simulink library "DriftControllerLibrary"  (R2014a)
settings: Solver=ode45  StartTime=0.0  StopTime=10.0  RelTol=1e-3
values from neighbouring files (symbols this model uses):
  alpha_lookup = alpha_sl:-0.001:-1*alpha_sl    [Fyf_lookup_table.m]
  alpha_prm = 0.9    [InitMap.m]
  beta_prm = 1    [InitMap.m]
  curve_prm = curve_prm.data    [InitMap.m]
  discrete_prm = discrete_prm.data    [InitMap.m]
  errLim_prm = 0.005    [InitMap.m]
  Fyf_lookup_2W = -Cf*tan(alpha_lookup) + Cf^2*(2 - mu_s_assumed_f/mu_p_assumed_f)*abs(tan(alpha_lookup)).*tan(alpha_lookup)/(3*mu_p_assumed_f*Fzf) -      Cf^3*tan(alpha_lookup).^3*(1-2*mu_s_assumed_f/(3*mu_p_assumed_f))/(9*mu_p_assumed_f^2*Fzf^2)    [Fyf_lookup_table.m]
  Fyf_lookup_4W = -(Cf/2)*tan(alpha_lookup) + (Cf/2)^2*(2 - mu_s_assumed_f/mu_p_assumed_f)*abs(tan(alpha_lookup)).*tan(alpha_lookup)/(3*mu_p_assumed_f*(Fzf/2)) -      (Cf/2)^3*tan(alpha_lookup).^3*(1-2*mu_s_assumed_f/(3*mu_p_assumed_f))/(9*mu_p_assumed_f^2*(Fzf/2)^2)    [Fyf_lookup_table.m]
  iterLim_prm = 30    [InitMap.m]
  map_prm = map_prm.data    [InitMap.m]
  numTerms_prm = 10    [InitMap.m]
  seg_prm = seg_prm.data    [InitMap.m]
  Ts = 0.002    [DSC_Control_Analysis.m]    (also in DSC_Control_Analysis_Exp.m; DSC_Speed_Control_Analysis.m; EC_params_nissan.m; Ext_MPCPara.m = SSD.Ts)
  useZ_prm = 0    [InitMap.m]
undefined symbols (not defined in the file or in its folder): ack, axInit, beta_vec, betaDes, betaThreshold, delta_sol, deltaLimits, Feasible, Fxr_sol, FxrEq, Fyf_sat, Fyf_sol, Kbeta, Kr, KUx, KUx_Drift, mu_p_assumed, mu_s_assumed, param, r_vec, rThreshold, sr, steering_limit, tau_DK, tau_DSC, tHold, tLimits, Ux_vec, UxEq, UxLimits, VoltsToTorque, VoltsToTorqueRegen, wc
libraries: DriftControllerLibrary x2, simulink x1
(part 1 of 2)
settings Model: Creator=Administrator  LastModifiedBy=cbeal

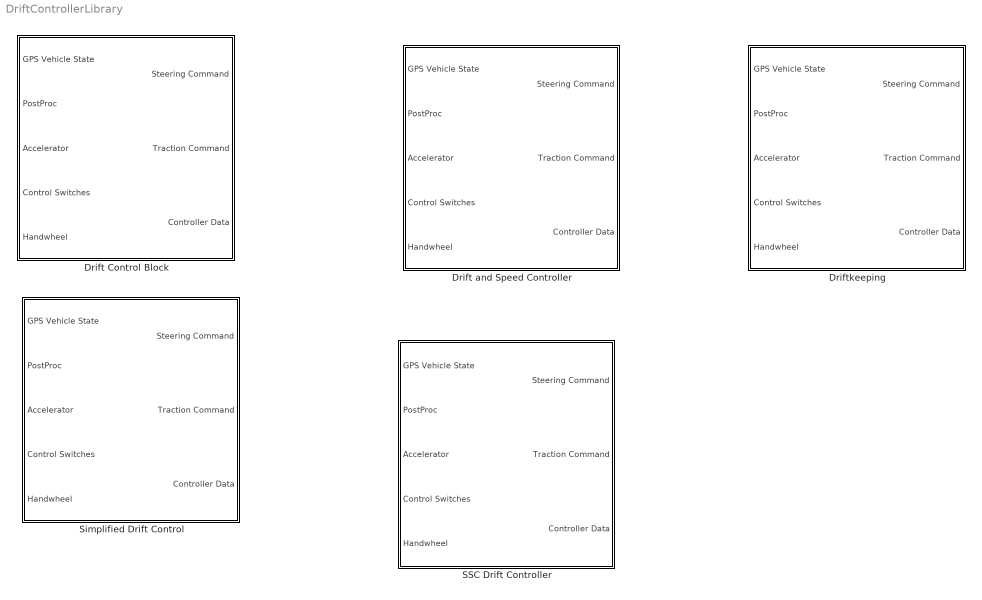
== system DriftControllerLibrary ==
  Drift Control Block : Subsystem  mask(Drift Controller Options){CoordinationEnable=on, UseGalvez=off, CoordType=Exact}
      mask prompts: CoordinationEnable "Use Longitudinal Coordination"; UseGalvez "Use Galvez Test Sequence"; CoordType "Coordination Method"
      mask init:
      | p1_params;
      | drift_params_DSC;
      | Fyf_lookup_table;
      | SteeringController;
      | 
      | coordinationswitch = [gcs '/Drift Control Block' '/Drift Controller Subsystem' '/Use Longitudinal Coordination'];
      | galvezswitch = [gcs '/Drift Control Block' '/Drift Controller Subsystem' '/Use Galvez Test Sequence'];
      | coordtypeswitch = [gcs '/Drift Control Block' '/Drift Controller Subsystem' '/Coordination Method'];
      | % NLObserverswitch = [gcs '/Nonlinear Observer' '/Enable Observer'];
      | % NLObserverStorageswitch = [gcs '/Nonlinear Observer' '/Enable Observer Estimate Storage'];
      | 
      | % default settings
      | set_param(coordinationswitch, 'value', '0');
      | set_param(galvezswitch, 'value', '0');
      | % set_param(NLObserverswitch, 'value', '1');
      | % set_param(NLObserverStorageswitch, 'value', '1'); 
      | 
      | %Look at checkbox to see if longitudinal coordination is desired
      | if (CoordinationEnable == 1)
      |     set_param(coordinationswitch, 'value', '1');
      | end
      | 
      | %Look at checkbox to see if Galvez test sequence is set
      | if (UseGalvez == 1)
      |     set_param(galvezswitch, 'value', '1');
      | end
      | 
      | %Look at popup menu to determine what coordination method to use
      | if (CoordType == 1)
      |     set_param(coordtypeswitch, 'value', '1');
      | elseif (CoordType == 2)
      |     set_param(coordtypeswitch, 'value', '2');
      | end
      mask TypeOptions CoordType: Linearization | Exact
  Drift and Speed Controller : Subsystem  mask(Drift Controller Options){UseGalvez=off}
      mask prompts: UseGalvez "Use Galvez Test Sequence"
      mask init:
      | p1_params;
      | drift_params_DSC_Speed;
      | SteeringController;
      | Fyf_lookup_table;
      | LoadDSCControlMap;
      | 
      | galvezswitch = [gcs '/Drift and Speed Controller' '/Drift Controller Subsystem' ...
      |     '/Use Galvez Test Sequence'];
      | 
      | % default settings
      | set_param(galvezswitch, 'value', '0');
      | 
      | %Look at checkbox to see if Galvez test sequence is set
      | if (UseGalvez == 1)
      |     set_param(galvezswitch, 'value', '1');
      | end
  Driftkeeping : Subsystem  mask(Drift Controller Options){}
      mask init:
      | p1_params;
      | driftkeeping_params;
      | Fyf_lookup_table;
      | SteeringController;
      | InitMap;
  SSC Drift Controller : Subsystem  mask(Drift Controller Options){UseGalvez=off}
      mask prompts: UseGalvez "Use Galvez Test Sequence"
      mask init:
      | p1_params;
      | drift_params_SSC;
      | SteeringController;
      | 
      | galvezswitch = [gcs '/SSC Drift Controller' '/SSC Drift Controller Subsystem' '/Use Galvez Test Sequence'];
      | % NLObserverswitch = [gcs '/Nonlinear Observer' '/Enable Observer'];
      | % NLObserverStorageswitch = [gcs '/Nonlinear Observer' '/Enable Observer Estimate Storage'];
      | 
      | % default settings
      | set_param(galvezswitch, 'value', '0');
      | % set_param(NLObserverswitch, 'value', '1');
      | % set_param(NLObserverStorageswitch, 'value', '1'); 
      | 
      | %Look at checkbox to see if Galvez test sequence is set
      | if (UseGalvez == 1)
      |     set_param(galvezswitch, 'value', '1');
      | end
  Simplified Drift Control : Subsystem  mask(Drift Controller Options){CoordinationEnable=Fxr, UseGalvez=off}
      mask prompts: CoordinationEnable "Use Longitudinal Coordination"; UseGalvez "Use Galvez Test Sequence"
      mask init:
      | p1_params;
      | drift_params_SDSC;
      | Fyf_lookup_table;
      | SteeringController;
      | 
      | coordinationswitch = [gcs '/Simplified Drift Control' '/Drift Controller Subsystem' '/Use Longitudinal Coordination'];
      | galvezswitch = [gcs '/Simplified Drift Control' '/Drift Controller Subsystem' '/Use Galvez Test Sequence'];
      | differentialswitch = [gcs '/Simplified Drift Control' '/Drift Controller Subsystem' '/Use Differential Drive'];
      | % NLObserverswitch = [gcs '/Nonlinear Observer' '/Enable Observer'];
      | % NLObserverStorageswitch = [gcs '/Nonlinear Observer' '/Enable Observer Estimate Storage'];
      | 
      | % default settings
      | set_param(coordinationswitch, 'value', '0');
      | set_param(galvezswitch, 'value', '0');
      | set_param(differentialswitch, 'value', '0');
      | % set_param(NLObserverswitch, 'value', '1');
      | % set_param(NLObserverStorageswitch, 'value', '1'); 
      | 
      | %Look at checkbox to see if longitudinal coordination is desired
      | if (CoordinationEnable == 2)
      |     set_param(coordinationswitch, 'value', '1');
      | end
      | 
      | if (CoordinationEnable == 3)
      |     set_param(differentialswitch, 'value', '1');
      | end
      | 
      | 
      | %Look at checkbox to see if Galvez test sequence is set
      | if (UseGalvez == 1)
      |     set_param(galvezswitch, 'value', '1');
      | end
      mask TypeOptions CoordinationEnable: None | Fxr | M_diff

== system DriftControllerLibrary/Drift Control Block ==
  GPS Vehicle State : Inport
  PostProc : Inport  Port=2
  Accelerator : Inport  Port=3
  Control Switches : Inport  Port=4
  Handwheel : Inport  Port=5
  Bus Selector1 : BusSelector  OutputSignals=Cruise Control Switch,Auto-Steer Switch,Brake Pedal Signal
  Drift Controller Subsystem : Subsystem
  Enable Logic : Subsystem
  Logical Operator : Logic  AllPortsSameDT=off  OutDataTypeStr=boolean
  Steering Command : Outport
  Traction Command : Outport  Port=2
  Controller Data : Outport  Port=3
  wires:
  Drift Controller Subsystem/3(Traction Command (A)) -> Traction Command/1
  Drift Controller Subsystem/2("Steering Command (rad, roadwheels)") -> Steering Command/1
  Drift Controller Subsystem/1(Controller Data) -> Controller Data/1
  Handwheel/1 -> Drift Controller Subsystem/3(Handwheel Angle)
  Accelerator/1 -> Drift Controller Subsystem/4(Go Pedal)
  GPS Vehicle State/1 -> Drift Controller Subsystem/2(GPS Vehicle State)
  PostProc/1 -> Drift Controller Subsystem/5(PostProc)
  Control Switches/1 -> Bus Selector1/1
  Enable Logic/1(Enable) -> Drift Controller Subsystem/1(Enable)
  Bus Selector1/1 -> Logical Operator/1  "<Cruise Control Switch>"
  Bus Selector1/2 -> Logical Operator/2  "<Auto-Steer Switch>"
  Bus Selector1/3 -> Enable Logic/2(Brake Pedal)  "<Brake Pedal Signal>"
  Logical Operator/1 -> Enable Logic/1(Enable Command)

== system DriftControllerLibrary/Drift and Speed Controller ==
  GPS Vehicle State : Inport
  PostProc : Inport  Port=2
  Accelerator : Inport  Port=3
  Control Switches : Inport  Port=4
  Handwheel : Inport  Port=5
  Bus Selector1 : BusSelector  OutputSignals=Cruise Control Switch,Auto-Steer Switch,Brake Pedal Signal
  Drift Controller Subsystem : Subsystem
  Enable Logic : Subsystem
  Logical Operator : Logic  AllPortsSameDT=off  OutDataTypeStr=boolean
  Steering Command : Outport
  Traction Command : Outport  Port=2
  Controller Data : Outport  Port=3
  wires:
  Logical Operator/1 -> Enable Logic/1(Enable Command)
  Bus Selector1/3 -> Enable Logic/2(Brake Pedal)  "<Brake Pedal Signal>"
  Bus Selector1/2 -> Logical Operator/2  "<Auto-Steer Switch>"
  Bus Selector1/1 -> Logical Operator/1  "<Cruise Control Switch>"
  Enable Logic/1(Enable) -> Drift Controller Subsystem/1(Enable)
  Control Switches/1 -> Bus Selector1/1
  PostProc/1 -> Drift Controller Subsystem/5(PostProc)
  GPS Vehicle State/1 -> Drift Controller Subsystem/2(GPS Vehicle State)
  Accelerator/1 -> Drift Controller Subsystem/4(Go Pedal)
  Handwheel/1 -> Drift Controller Subsystem/3(Handwheel Angle)
  Drift Controller Subsystem/1(Controller Data) -> Controller Data/1
  Drift Controller Subsystem/2("Steering Command (rad, roadwheels)") -> Steering Command/1
  Drift Controller Subsystem/3(Traction Command (A)) -> Traction Command/1

== system DriftControllerLibrary/Driftkeeping ==
  GPS Vehicle State : Inport
  PostProc : Inport  Port=2
  Accelerator : Inport  Port=3
  Control Switches : Inport  Port=4
  Handwheel : Inport  Port=5
  Bus Selector1 : BusSelector  OutputSignals=Cruise Control Switch,Auto-Steer Switch,Brake Pedal Signal
  Driftkeeping Subsystem : Subsystem
  Enable Logic : Subsystem
  Logical Operator : Logic  AllPortsSameDT=off  OutDataTypeStr=boolean
  Steering Command : Outport
  Traction Command : Outport  Port=2
  Controller Data : Outport  Port=3
  wires:
  Logical Operator/1 -> Enable Logic/1(Enable Command)
  Bus Selector1/3 -> Enable Logic/2(Brake Pedal)  "<Brake Pedal Signal>"
  Bus Selector1/2 -> Logical Operator/2  "<Auto-Steer Switch>"
  Bus Selector1/1 -> Logical Operator/1  "<Cruise Control Switch>"
  Enable Logic/1(Enable) -> Driftkeeping Subsystem/1(Enable)
  Control Switches/1 -> Bus Selector1/1
  PostProc/1 -> Driftkeeping Subsystem/5(PostProc)
  GPS Vehicle State/1 -> Driftkeeping Subsystem/2(GPS Vehicle State)
  Accelerator/1 -> Driftkeeping Subsystem/4(Go Pedal)
  Handwheel/1 -> Driftkeeping Subsystem/3(Handwheel Angle)
  Driftkeeping Subsystem/1(Controller Data) -> Controller Data/1
  Driftkeeping Subsystem/2("Steering Command (rad, roadwheels)") -> Steering Command/1
  Driftkeeping Subsystem/3(Traction Command (A)) -> Traction Command/1

== system DriftControllerLibrary/SSC Drift Controller ==
  GPS Vehicle State : Inport
  PostProc : Inport  Port=2
  Accelerator : Inport  Port=3
  Control Switches : Inport  Port=4
  Handwheel : Inport  Port=5
  Bus Selector1 : BusSelector  OutputSignals=Cruise Control Switch,Auto-Steer Switch,Brake Pedal Signal
  Enable Logic : Subsystem
  Logical Operator : Logic  AllPortsSameDT=off  OutDataTypeStr=boolean
  SSC Drift Controller Subsystem : Subsystem
  Terminator : Terminator
  Steering Command : Outport
  Traction Command : Outport  Port=2
  Controller Data : Outport  Port=3
  wires:
  Logical Operator/1 -> Enable Logic/1(Enable Command)
  Bus Selector1/3 -> Enable Logic/2(Brake Pedal)  "<Brake Pedal Signal>"
  Bus Selector1/2 -> Logical Operator/2  "<Auto-Steer Switch>"
  Bus Selector1/1 -> Logical Operator/1  "<Cruise Control Switch>"
  Enable Logic/1(Enable) -> SSC Drift Controller Subsystem/1(Enable)
  Control Switches/1 -> Bus Selector1/1
  GPS Vehicle State/1 -> SSC Drift Controller Subsystem/2(GPS Vehicle State)
  Accelerator/1 -> SSC Drift Controller Subsystem/4(Go Pedal)
  Handwheel/1 -> SSC Drift Controller Subsystem/3(Handwheel Angle)
  SSC Drift Controller Subsystem/1(Controller Data) -> Controller Data/1
  SSC Drift Controller Subsystem/2("Steering Command (rad, roadwheels)") -> Steering Command/1
  SSC Drift Controller Subsystem/3(Traction Command (A)) -> Traction Command/1
  PostProc/1 -> Terminator/1

== system DriftControllerLibrary/Simplified Drift Control ==
  GPS Vehicle State : Inport
  PostProc : Inport  Port=2
  Accelerator : Inport  Port=3
  Control Switches : Inport  Port=4
  Handwheel : Inport  Port=5
  Bus Selector1 : BusSelector  OutputSignals=Cruise Control Switch,Auto-Steer Switch,Brake Pedal Signal
  Drift Controller Subsystem : Subsystem
  Enable Logic : Subsystem
  Logical Operator : Logic  AllPortsSameDT=off  OutDataTypeStr=boolean
  Steering Command : Outport
  Traction Command : Outport  Port=2
  Controller Data : Outport  Port=3
  wires:
  Drift Controller Subsystem/3(Traction Command (A)) -> Traction Command/1
  Drift Controller Subsystem/2("Steering Command (rad, roadwheels)") -> Steering Command/1
  Drift Controller Subsystem/1(Controller Data) -> Controller Data/1
  Handwheel/1 -> Drift Controller Subsystem/3(Handwheel Angle)
  Accelerator/1 -> Drift Controller Subsystem/4(Go Pedal)
  GPS Vehicle State/1 -> Drift Controller Subsystem/2(GPS Vehicle State)
  PostProc/1 -> Drift Controller Subsystem/5(PostProc)
  Control Switches/1 -> Bus Selector1/1
  Enable Logic/1(Enable) -> Drift Controller Subsystem/1(Enable)
  Bus Selector1/1 -> Logical Operator/1  "<Cruise Control Switch>"
  Bus Selector1/2 -> Logical Operator/2  "<Auto-Steer Switch>"
  Bus Selector1/3 -> Enable Logic/2(Brake Pedal)  "<Brake Pedal Signal>"
  Logical Operator/1 -> Enable Logic/1(Enable Command)

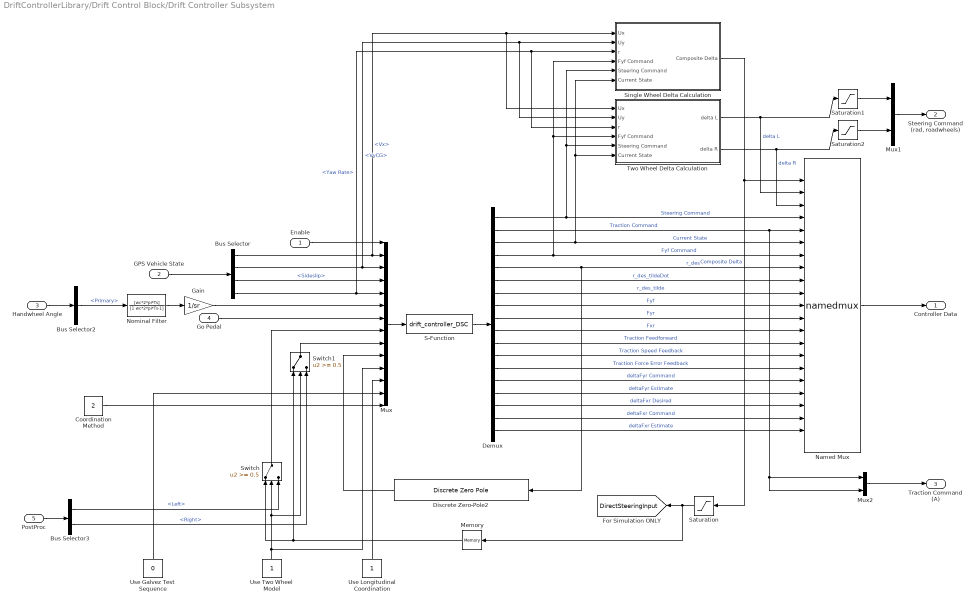
== system DriftControllerLibrary/Drift Control Block/Drift Controller Subsystem ==
  Enable : Inport
  GPS Vehicle State : Inport  Port=2
  Handwheel Angle : Inport  Port=3
  Go Pedal : Inport  Port=4
  PostProc : Inport  Port=5
  Bus Selector : BusSelector  OutputSignals=Vx,VyCG,Sideslip,Yaw Rate
  Bus Selector2 : BusSelector  OutputSignals=Primary
  Bus Selector3 : BusSelector  OutputSignals=Steer Angles.Left,Steer Angles.Right
  Coordination Method : Constant  Value=2
  Demux : Demux  Outputs=18
  Discrete Zero-Pole2 : DiscreteZeroPole  Zeros=[]  Poles=[exp(-Ts/tau_DSC)]  Gain=1-exp(-Ts/tau_DSC)  SampleTime=Ts
  Gain : Gain  Gain=1/sr
  Memory : Memory
  Mux : Mux  Inputs=14
  Mux1 : Mux  Inputs=2
  Mux2 : Mux  Inputs=2
  Named Mux : S-Function  FunctionName=namedmux  Parameters=inputcount,inputsizes  EnableBusSupport=off  mask{fname=datadescDriftController}
      mask prompts: fname "Data description function name"
      mask help:
      | Combines input signals into a single output vector, according to a structure that provides the names and sizes of each signal.
      |
      | The parameter below should be set to the name of a function which returns a 1xN structure array, where N is the number of input signals.  The structure should contain fields "size" which specifies the width of the input signal, and "name" which specifies its name.
      mask init:
      | desc=eval(fname);
      | %if(class(desc)~='cell')
      | %	error('Incorrect description');
      | %end
      | inputcount=length(desc);
      | if((inputcount<1)|(inputcount>50))
      | 	error('Inappropriate number of inputs.');
      | end
      | 
      | inputsizes=[desc.size];
      | 
      | x=min(inputcount*ones(1,50),1:50);
      mask Display:
      | port_label('input',x(1),desc(x(1)).name);
      | port_label('input',x(2),desc(x(2)).name);
      | port_label('input',x(3),desc(x(3)).name);
      | port_label('input',x(4),desc(x(4)).name);
      | port_label('input',x(5),desc(x(5)).name);
      | port_label('input',x(6),desc(x(6)).name);
      | port_label('input',x(7),desc(x(7)).name);
      | port_label('input',x(8),desc(x(8)).name);
      | port_label('input',x(9),desc(x(9)).name);
      | port_label('input',x(10),desc(x(10)).name);
      | port_label('input',x(11),desc(x(11)).name);
      | port_label('input',x(12),desc(x(12)).name);
      | port_label('input',x(13),desc(x(13)).name);
      | port_label('input',x(14),desc(x(14)).name);
      | port_label('input',x(15),desc(x(15)).name);
      | port_label('input',x(16),desc(x(16)).name);
      | port_label('input',x(17),desc(x(17)).name);
      | port_label('input',x(18),desc(x(18)).name);
      | port_label('input',x(19),desc(x(19)).name);
      | port_label('input',x(20),desc(x(20)).name);
      | port_label('input',x(21),desc(x(21)).name);
      | port_label('input',x(22),desc(x(22)).name);
      | port_label('input',x(23),desc(x(23)).name);
      | port_label('input',x(24),desc(x(24)).name);
      | port_label('input',x(25),desc(x(25)).name);
      | port_label('input',x(26),desc(x(26)).name);
      | port_label('input',x(27),desc(x(27)).name);
      | port_label('input',x(28),desc(x(28)).name);
      | port_label('input',x(29),desc(x(29)).name);
      | port_label('input',x(30),desc(x(30)).name);
  Nominal Filter : DiscreteFilter  Numerator=[wc*2*pi*Ts]  Denominator=[1 wc*2*pi*Ts-1]  SampleTime=Ts
  S-Function : S-Function  FunctionName=drift_controller_DSC  Parameters=axInit,tHold,UxLimits,deltaLimits,tLimits,betaThreshold,rThreshold,betaDes,UxEq,FxrEq,Kbeta,Kr,KUx,KUx_Drift,tau_DSC,VoltsToTorque,VoltsToTorqueRegen,param.drive_ratio,param.rl.r,param.m,param.Iz,param.a,param.b,param.c,param.fl.C,param.fr.C,param.rl.C,param.rr.C,mu_p_assumed,mu_s_assumed,Fyf_sat,Ts  EnableBusSupport=off
  Saturation : Saturate  UpperLimit=steering_limit*pi/180  LowerLimit=-steering_limit*pi/180
  Saturation1 : Saturate  UpperLimit=steering_limit*pi/180  LowerLimit=-steering_limit*pi/180
  Saturation2 : Saturate  UpperLimit=steering_limit*pi/180  LowerLimit=-steering_limit*pi/180
  Single Wheel Delta Calculation : Subsystem
  Switch : Switch  Threshold=0.5
  Switch1 : Switch  Threshold=0.5
  Two Wheel Delta Calculation : Subsystem
  Use Galvez Test Sequence : Constant  Value=0
  Use Longitudinal Coordination : Constant
  Use Two Wheel Model : Constant
  Controller Data : Outport
  "Steering Command (rad, roadwheels)" : Outport  Port=2
  Traction Command (A) : Outport  Port=3
  tag scope: DirectSteeringInput=global
  wires:
  Coordination Method/1 -> Mux/14
  Mux2/1 -> Traction Command (A)/1
  Nominal Filter/1 -> Gain/1
  Bus Selector2/1 -> Nominal Filter/1  "<Primary>"
  Demux/14 -> Named Mux/17  "deltaFyr Command"
  Single Wheel Delta Calculation/1(Composite Delta) -> Saturation/1, Named Mux/1  "Composite Delta"
  Demux/1 -> Single Wheel Delta Calculation/5(Steering Command), Two Wheel Delta Calculation/5(Steering Command), Named Mux/4  "Steering Command"
  Demux/2 -> Mux2/2, Mux2/1, Named Mux/5  "Traction Command"
  Demux/3 -> Single Wheel Delta Calculation/6(Current State), Two Wheel Delta Calculation/6(Current State), Named Mux/6  "Current State"
  Demux/5 -> Discrete Zero-Pole2/1, Named Mux/8  "r_des"
  Demux/4 -> Single Wheel Delta Calculation/4(Fyf Command), Two Wheel Delta Calculation/4(Fyf Command), Named Mux/7  "Fyf Command"
  Named Mux/1 -> Controller Data/1
  Demux/18 -> Named Mux/21  "deltaFxr Estimate"
  Demux/17 -> Named Mux/20  "deltaFxr Command"
  Demux/16 -> Named Mux/19  "deltaFxr Desired"
  Demux/15 -> Named Mux/18  "deltaFyr Estimate"
  Demux/13 -> Named Mux/16  "Traction Force Error Feedback"
  Demux/12 -> Named Mux/15  "Traction Speed Feedback"
  Demux/11 -> Named Mux/14  "Traction Feedforward"
  Demux/10 -> Named Mux/13  "Fxr"
  Demux/9 -> Named Mux/12  "Fyr"
  Demux/8 -> Named Mux/11  "Fyf"
  Demux/7 -> Named Mux/10  "r_des_tilde"
  Demux/6 -> Named Mux/9  "r_des_tildeDot"
  Two Wheel Delta Calculation/2(delta R) -> Named Mux/3, Saturation2/1  "delta R"
  Saturation2/1 -> Mux1/2
  Saturation1/1 -> Mux1/1
  Mux1/1 -> "Steering Command (rad, roadwheels)"/1
  Enable/1 -> Mux/1
  Use Galvez Test Sequence/1 -> Mux/13
  Use Longitudinal Coordination/1 -> Mux/12
  Discrete Zero-Pole2/1 -> Mux/10
  Switch1/1 -> Mux/9
  Switch/1 -> Mux/8
  Use Two Wheel Model/1 -> Mux/11, Switch/2, Switch1/2
  Bus Selector3/2 -> Switch1/3  "<Right>"
  Bus Selector3/1 -> Switch/3  "<Left>"
  Memory/1 -> Switch1/1, Switch/1
  Two Wheel Delta Calculation/1(delta L) -> Named Mux/2, Saturation1/1  "delta L"
  Saturation/1 -> Memory/1, [DirectSteeringInput]
  PostProc/1 -> Bus Selector3/1
  Bus Selector/4 -> Two Wheel Delta Calculation/3(r), Single Wheel Delta Calculation/3(r), Mux/5  "<Yaw Rate>"
  Bus Selector/3 -> Mux/4  "<Sideslip>"
  Bus Selector/2 -> Two Wheel Delta Calculation/2(Uy), Single Wheel Delta Calculation/2(Uy), Mux/3  "<VyCG>"
  Gain/1 -> Mux/6
  Go Pedal/1 -> Mux/7
  Mux/1 -> S-Function/1
  Bus Selector/1 -> Two Wheel Delta Calculation/1(Ux), Single Wheel Delta Calculation/1(Ux), Mux/2  "<Vx>"
  S-Function/1 -> Demux/1
  Handwheel Angle/1 -> Bus Selector2/1
  GPS Vehicle State/1 -> Bus Selector/1

== system DriftControllerLibrary/Drift Control Block/Enable Logic ==
  Enable Command : Inport
  Brake Pedal : Inport  Port=2
  Delay : Subsystem
  Latch1 : Subsystem  TreatAsAtomicUnit=on
  Logical Operator : Logic  Operator=OR  AllPortsSameDT=off  OutDataTypeStr=float('double')
  Logical Operator1 : Logic  AllPortsSameDT=off  OutDataTypeStr=float('double')
  Logical Operator2 : Logic  Operator=NOT  AllPortsSameDT=off  OutDataTypeStr=float('double')
  Enable : Outport
  wires:
  Logical Operator2/1 -> Logical Operator1/2
  Logical Operator1/1 -> Latch1/1(In1)
  Logical Operator/1 -> Latch1/Trigger
  Brake Pedal/1 -> Logical Operator/2, Logical Operator2/1
  Delay/1(Out) -> Logical Operator/1
  Enable Command/1 -> Logical Operator1/1, Delay/1(In)
  Latch1/1(Out1) -> Enable/1

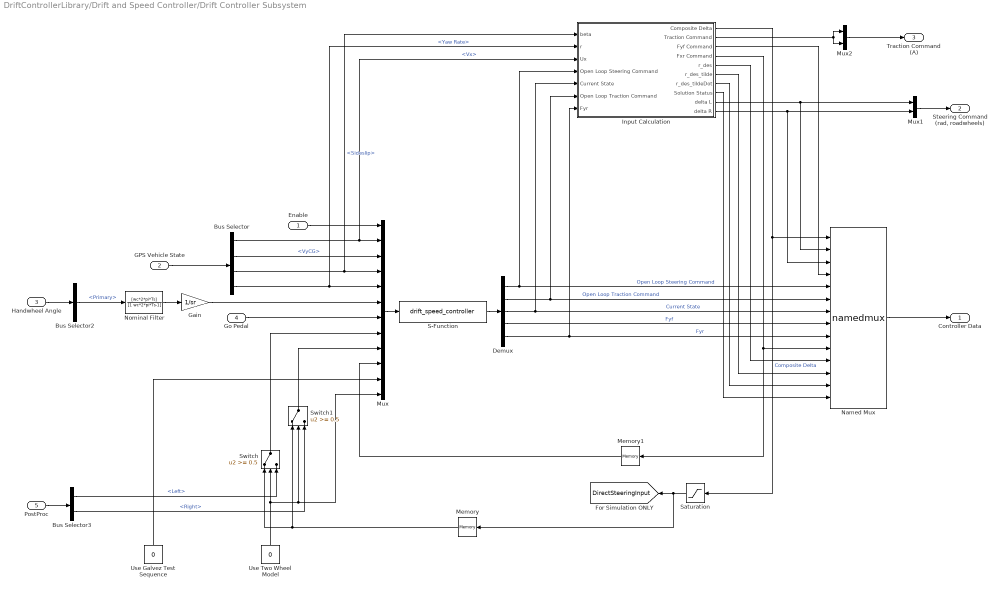
== system DriftControllerLibrary/Drift and Speed Controller/Drift Controller Subsystem ==
  Enable : Inport
  GPS Vehicle State : Inport  Port=2
  Handwheel Angle : Inport  Port=3
  Go Pedal : Inport  Port=4
  PostProc : Inport  Port=5
  Bus Selector : BusSelector  OutputSignals=Vx,VyCG,Sideslip,Yaw Rate
  Bus Selector2 : BusSelector  OutputSignals=Primary
  Bus Selector3 : BusSelector  OutputSignals=Steer Angles.Left,Steer Angles.Right
  Demux : Demux  Outputs=5
  Gain : Gain  Gain=1/sr
  Input Calculation : Subsystem
  Memory : Memory
  Memory1 : Memory
  Mux : Mux  Inputs=12
  Mux1 : Mux  Inputs=2
  Mux2 : Mux  Inputs=2
  Named Mux : S-Function  FunctionName=namedmux  Parameters=inputcount,inputsizes  EnableBusSupport=off  mask{fname=datadescDriftSpeedController}
      mask prompts: fname "Data description function name"
      mask help:
      | Combines input signals into a single output vector, according to a structure that provides the names and sizes of each signal.
      |
      | The parameter below should be set to the name of a function which returns a 1xN structure array, where N is the number of input signals.  The structure should contain fields "size" which specifies the width of the input signal, and "name" which specifies its name.
      mask init: same as DriftControllerLibrary/Drift Control Block/Drift Controller Subsystem/Named Mux
      mask Display:
      | port_label('input',x(1),desc(x(1)).name);
      | port_label('input',x(2),desc(x(2)).name);
      | port_label('input',x(3),desc(x(3)).name);
      | port_label('input',x(4),desc(x(4)).name);
      | port_label('input',x(5),desc(x(5)).name);
      | port_label('input',x(6),desc(x(6)).name);
      | port_label('input',x(7),desc(x(7)).name);
      | port_label('input',x(8),desc(x(8)).name);
      | port_label('input',x(9),desc(x(9)).name);
      | port_label('input',x(10),desc(x(10)).name);
      | port_label('input',x(11),desc(x(11)).name);
      | port_label('input',x(12),desc(x(12)).name);
      | port_label('input',x(13),desc(x(13)).name);
      | port_label('input',x(14),desc(x(14)).name);
      | port_label('input',x(15),desc(x(15)).name);
      | port_label('input',x(16),desc(x(16)).name);
      | port_label('input',x(17),desc(x(17)).name);
      | port_label('input',x(18),desc(x(18)).name);
      | port_label('input',x(19),desc(x(19)).name);
      | port_label('input',x(20),desc(x(20)).name);
      | port_label('input',x(21),desc(x(21)).name);
      | port_label('input',x(22),desc(x(22)).name);
      | port_label('input',x(23),desc(x(23)).name);
      | port_label('input',x(24),desc(x(24)).name);
      | port_label('input',x(25),desc(x(25)).name);
      | port_label('input',x(26),desc(x(26)).name);
      | port_label('input',x(27),desc(x(27)).name);
      | port_label('input',x(28),desc(x(28)).name);
      | port_label('input',x(29),desc(x(29)).name);
      | port_label('input',x(30),desc(x(30)).name);
  Nominal Filter : DiscreteFilter  Numerator=[wc*2*pi*Ts]  Denominator=[1 wc*2*pi*Ts-1]  SampleTime=Ts
  S-Function : S-Function  FunctionName=drift_speed_controller  Parameters=axInit,tHold,UxLimits,deltaLimits,tLimits, KUx, betaThreshold,rThreshold,VoltsToTorque,VoltsToTorqueRegen,param.drive_ratio,param.rl.r,param.m,param.Iz,param.a,param.b,param.c,param.fl.C,param.fr.C,param.rl.C,param.rr.C,mu_p_assumed,mu_s_assumed,Ts  EnableBusSupport=off
  Saturation : Saturate  UpperLimit=steering_limit*pi/180  LowerLimit=-steering_limit*pi/180
  Switch : Switch  Threshold=0.5
  Switch1 : Switch  Threshold=0.5
  Use Galvez Test Sequence : Constant  Value=0
  Use Two Wheel Model : Constant  Value=0
  Controller Data : Outport
  "Steering Command (rad, roadwheels)" : Outport  Port=2
  Traction Command (A) : Outport  Port=3
  tag scope: DirectSteeringInput=global
  wires:
  GPS Vehicle State/1 -> Bus Selector/1
  Handwheel Angle/1 -> Bus Selector2/1
  Bus Selector/1 -> Mux/2, Input Calculation/3(Ux)  "<Vx>"
  Mux/1 -> S-Function/1
  Go Pedal/1 -> Mux/7
  Gain/1 -> Mux/6
  Bus Selector/2 -> Mux/3  "<VyCG>"
  Bus Selector/3 -> Mux/4, Input Calculation/1(beta)  "<Sideslip>"
  Bus Selector/4 -> Mux/5, Input Calculation/2(r)  "<Yaw Rate>"
  PostProc/1 -> Bus Selector3/1
  Saturation/1 -> [DirectSteeringInput], Memory/1
  Memory/1 -> Switch/1, Switch1/1
  Bus Selector3/1 -> Switch/3  "<Left>"
  Bus Selector3/2 -> Switch1/3  "<Right>"
  Use Two Wheel Model/1 -> Switch/2, Switch1/2, Mux/12
  Switch/1 -> Mux/8
  Switch1/1 -> Mux/9
  Enable/1 -> Mux/1
  Mux1/1 -> "Steering Command (rad, roadwheels)"/1
  Named Mux/1 -> Controller Data/1
  Demux/3 -> Input Calculation/5(Current State), Named Mux/7  "Current State"
  Input Calculation/1(Composite Delta) -> Saturation/1, Named Mux/1  "Composite Delta"
  Bus Selector2/1 -> Nominal Filter/1  "<Primary>"
  Nominal Filter/1 -> Gain/1
  Demux/2 -> Input Calculation/6(Open Loop Traction Command), Named Mux/6  "Open Loop Traction Command"
  Mux2/1 -> Traction Command (A)/1
  Input Calculation/2(Traction Command) -> Mux2/1, Mux2/2
  S-Function/1 -> Demux/1
  Demux/1 -> Named Mux/5, Input Calculation/4(Open Loop Steering Command)  "Open Loop Steering Command"
  Input Calculation/3(Fyf Command) -> Named Mux/4
  Demux/4 -> Named Mux/8  "Fyf"
  Demux/5 -> Named Mux/9, Input Calculation/7(Fyr)  "Fyr"
  Input Calculation/5(r_des) -> Named Mux/11
  Input Calculation/6(r_des_tilde) -> Named Mux/12
  Input Calculation/7(r_des_tildeDot) -> Named Mux/13
  Input Calculation/4(Fxr Command) -> Named Mux/10, Memory1/1
  Input Calculation/8(Solution Status) -> Named Mux/14
  Use Galvez Test Sequence/1 -> Mux/11
  Memory1/1 -> Mux/10
  Input Calculation/9(delta L) -> Named Mux/2, Mux1/1
  Input Calculation/10(delta R) -> Named Mux/3, Mux1/2

== system DriftControllerLibrary/Drift and Speed Controller/Enable Logic ==
  Enable Command : Inport
  Brake Pedal : Inport  Port=2
  Delay : Subsystem
  Latch1 : Subsystem  TreatAsAtomicUnit=on
  Logical Operator : Logic  Operator=OR  AllPortsSameDT=off  OutDataTypeStr=float('double')
  Logical Operator1 : Logic  AllPortsSameDT=off  OutDataTypeStr=float('double')
  Logical Operator2 : Logic  Operator=NOT  AllPortsSameDT=off  OutDataTypeStr=float('double')
  Enable : Outport
  wires:
  Latch1/1(Out1) -> Enable/1
  Enable Command/1 -> Delay/1(In), Logical Operator1/1
  Delay/1(Out) -> Logical Operator/1
  Brake Pedal/1 -> Logical Operator2/1, Logical Operator/2
  Logical Operator/1 -> Latch1/Trigger
  Logical Operator1/1 -> Latch1/1(In1)
  Logical Operator2/1 -> Logical Operator1/2

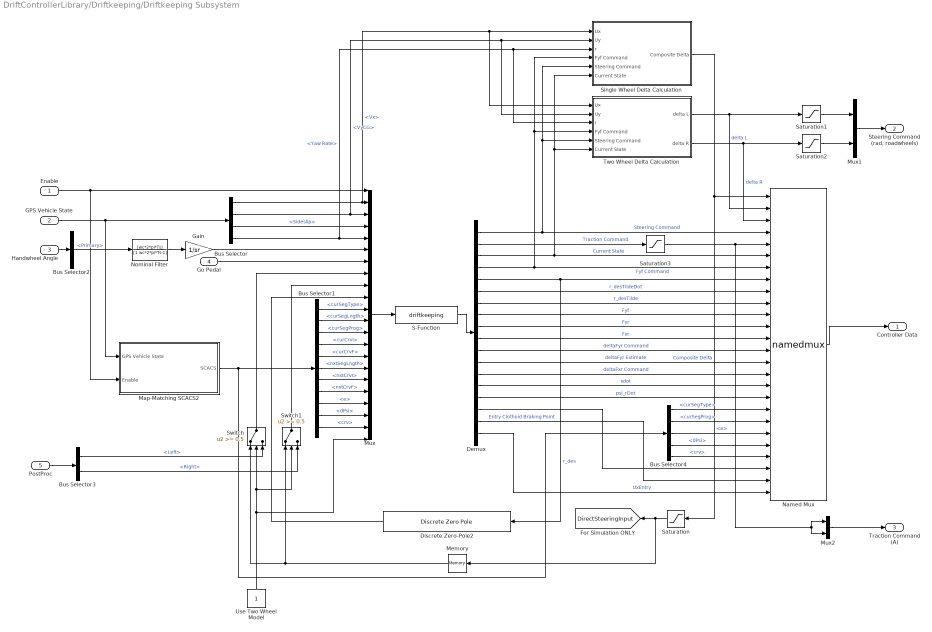
== system DriftControllerLibrary/Driftkeeping/Driftkeeping Subsystem ==
  Enable : Inport
  GPS Vehicle State : Inport  Port=2
  Handwheel Angle : Inport  Port=3
  Go Pedal : Inport  Port=4
  PostProc : Inport  Port=5
  Bus Selector : BusSelector  OutputSignals=Vx,VyCG,Sideslip,Yaw Rate
  Bus Selector1 : BusSelector  OutputSignals=curOut.curSegType,curOut.curSegLngth,curOut.curSegProg,curOut.curCrvI,curOut.curCrvF,nxtOut.nxtSegLngth,nxtOut.nxtCrvI,nxtOut.nxtCrvF,matchOut.e,matchOut.dPsi,matchOut.crv
  Bus Selector2 : BusSelector  OutputSignals=Primary
  Bus Selector3 : BusSelector  OutputSignals=Steer Angles.Left,Steer Angles.Right
  Bus Selector4 : BusSelector  OutputSignals=curOut.curSegType,curOut.curSegProg,matchOut.e,matchOut.dPsi,matchOut.crv
  Demux : Demux  Outputs=18
  Discrete Zero-Pole2 : DiscreteZeroPole  Zeros=[]  Poles=[exp(-Ts/tau_DK)]  Gain=1-exp(-Ts/tau_DK)  SampleTime=Ts
  Gain : Gain  Gain=1/sr
  Map-Matching SCACS2 : Subsystem
  Memory : Memory
  Mux : Mux  Inputs=22
  Mux1 : Mux  Inputs=2
  Mux2 : Mux  Inputs=2
  Named Mux : S-Function  FunctionName=namedmux  Parameters=inputcount,inputsizes  EnableBusSupport=off  mask{fname=datadescDriftkeeping}
      mask prompts: fname "Data description function name"
      mask help:
      | Combines input signals into a single output vector, according to a structure that provides the names and sizes of each signal.
      |
      | The parameter below should be set to the name of a function which returns a 1xN structure array, where N is the number of input signals.  The structure should contain fields "size" which specifies the width of the input signal, and "name" which specifies its name.
      mask init: same as DriftControllerLibrary/Drift Control Block/Drift Controller Subsystem/Named Mux
      mask Display:
      | port_label('input',x(1),desc(x(1)).name);
      | port_label('input',x(2),desc(x(2)).name);
      | port_label('input',x(3),desc(x(3)).name);
      | port_label('input',x(4),desc(x(4)).name);
      | port_label('input',x(5),desc(x(5)).name);
      | port_label('input',x(6),desc(x(6)).name);
      | port_label('input',x(7),desc(x(7)).name);
      | port_label('input',x(8),desc(x(8)).name);
      | port_label('input',x(9),desc(x(9)).name);
      | port_label('input',x(10),desc(x(10)).name);
      | port_label('input',x(11),desc(x(11)).name);
      | port_label('input',x(12),desc(x(12)).name);
      | port_label('input',x(13),desc(x(13)).name);
      | port_label('input',x(14),desc(x(14)).name);
      | port_label('input',x(15),desc(x(15)).name);
      | port_label('input',x(16),desc(x(16)).name);
      | port_label('input',x(17),desc(x(17)).name);
      | port_label('input',x(18),desc(x(18)).name);
      | port_label('input',x(19),desc(x(19)).name);
      | port_label('input',x(20),desc(x(20)).name);
      | port_label('input',x(21),desc(x(21)).name);
      | port_label('input',x(22),desc(x(22)).name);
      | port_label('input',x(23),desc(x(23)).name);
      | port_label('input',x(24),desc(x(24)).name);
      | port_label('input',x(25),desc(x(25)).name);
      | port_label('input',x(26),desc(x(26)).name);
      | port_label('input',x(27),desc(x(27)).name);
      | port_label('input',x(28),desc(x(28)).name);
      | port_label('input',x(29),desc(x(29)).name);
      | port_label('input',x(30),desc(x(30)).name);
  Nominal Filter : DiscreteFilter  Numerator=[wc*2*pi*Ts]  Denominator=[1 wc*2*pi*Ts-1]  SampleTime=Ts
  S-Function : S-Function  FunctionName=driftkeeping  Parameters=KUx, UxEntryScaleFactor, UxConst, UxExit, xla, Ke, Kr, tau_DK, VoltsToTorque,VoltsToTorqueRegen,param.drive_ratio,param.rl.r,param.m,param.Iz,param.a,param.b,param.c,param.fl.C,param.fr.C,param.rl.C,param.rr.C,mu_p_assumed_f,mu_s_assumed_f,mu_p_assumed_r,mu_s_assumed_r,Fyf_sat,Ts  EnableBusSupport=off
  Saturation : Saturate  UpperLimit=steering_limit*pi/180  LowerLimit=-steering_limit*pi/180
  Saturation1 : Saturate  UpperLimit=steering_limit*pi/180  LowerLimit=-steering_limit*pi/180
  Saturation2 : Saturate  UpperLimit=steering_limit*pi/180  LowerLimit=-steering_limit*pi/180
  Saturation3 : Saturate  UpperLimit=2.8  LowerLimit=0.9
  Single Wheel Delta Calculation : Subsystem
  Switch : Switch  Threshold=0.5
  Switch1 : Switch  Threshold=0.5
  Two Wheel Delta Calculation : Subsystem
  Use Two Wheel Model : Constant
  Controller Data : Outport
  "Steering Command (rad, roadwheels)" : Outport  Port=2
  Traction Command (A) : Outport  Port=3
  tag scope: DirectSteeringInput=global
  wires:
  Demux/18 -> Named Mux/26  "UxEntry"
  Demux/17 -> Named Mux/25  "Entry Clothoid Braking Point"
  Demux/16 -> Named Mux/24
  Bus Selector1/11 -> Mux/21  "<crv>"
  Bus Selector1/10 -> Mux/20  "<dPsi>"
  Bus Selector1/9 -> Mux/19  "<e>"
  Bus Selector1/8 -> Mux/18  "<nxtCrvF>"
  Bus Selector1/7 -> Mux/17  "<nxtCrvI>"
  Bus Selector1/6 -> Mux/16  "<nxtSegLngth>"
  Bus Selector1/5 -> Mux/15  "<curCrvF>"
  Bus Selector1/4 -> Mux/14  "<curCrvI>"
  Bus Selector1/3 -> Mux/13  "<curSegProg>"
  Bus Selector1/2 -> Mux/12  "<curSegLngth>"
  Bus Selector1/1 -> Mux/11  "<curSegType>"
  Handwheel Angle/1 -> Bus Selector2/1
  S-Function/1 -> Demux/1
  Bus Selector/1 -> Mux/2, Single Wheel Delta Calculation/1(Ux), Two Wheel Delta Calculation/1(Ux)  "<Vx>"
  Mux/1 -> S-Function/1
  Go Pedal/1 -> Mux/7
  Gain/1 -> Mux/6
  Bus Selector/2 -> Mux/3, Single Wheel Delta Calculation/2(Uy), Two Wheel Delta Calculation/2(Uy)  "<VyCG>"
  Bus Selector/3 -> Mux/4  "<Sideslip>"
  Bus Selector/4 -> Mux/5, Single Wheel Delta Calculation/3(r), Two Wheel Delta Calculation/3(r)  "<Yaw Rate>"
  PostProc/1 -> Bus Selector3/1
  Saturation/1 -> [DirectSteeringInput], Memory/1
  Two Wheel Delta Calculation/1(delta L) -> Saturation1/1, Named Mux/2  "delta L"
  Memory/1 -> Switch/1, Switch1/1
  Bus Selector3/1 -> Switch/3  "<Left>"
  Bus Selector3/2 -> Switch1/3  "<Right>"
  Use Two Wheel Model/1 -> Mux/22, Switch1/2, Switch/2
  Switch/1 -> Mux/8
  Switch1/1 -> Mux/9
  Discrete Zero-Pole2/1 -> Mux/10
  Enable/1 -> Mux/1, Map-Matching SCACS2/2(Enable)
  Mux1/1 -> "Steering Command (rad, roadwheels)"/1
  Saturation1/1 -> Mux1/1
  Saturation2/1 -> Mux1/2
  Two Wheel Delta Calculation/2(delta R) -> Saturation2/1, Named Mux/3  "delta R"
  Demux/6 -> Named Mux/9  "r_desTildeDot"
  Demux/7 -> Named Mux/10  "r_desTilde"
  Demux/8 -> Named Mux/11  "Fyf"
  Demux/9 -> Named Mux/12  "Fyr"
  Demux/10 -> Named Mux/13  "Fxr"
  Named Mux/1 -> Controller Data/1
  Demux/4 -> Named Mux/7, Two Wheel Delta Calculation/4(Fyf Command), Single Wheel Delta Calculation/4(Fyf Command)  "Fyf Command"
  Demux/5 -> Named Mux/8, Discrete Zero-Pole2/1  "r_des"
  Demux/3 -> Named Mux/6, Two Wheel Delta Calculation/6(Current State), Single Wheel Delta Calculation/6(Current State)  "Current State"
  Demux/1 -> Named Mux/4, Two Wheel Delta Calculation/5(Steering Command), Single Wheel Delta Calculation/5(Steering Command)  "Steering Command"
  Single Wheel Delta Calculation/1(Composite Delta) -> Named Mux/1, Saturation/1  "Composite Delta"
  Bus Selector2/1 -> Nominal Filter/1  "<Primary>"
  Nominal Filter/1 -> Gain/1
  Mux2/1 -> Traction Command (A)/1
  Demux/11 -> Named Mux/14  "deltaFyr Command"
  Demux/12 -> Named Mux/15  "deltaFyr Estimate"
  Demux/13 -> Named Mux/16  "deltaFxr Command"
  Demux/14 -> Named Mux/17  "sdot"
  Demux/15 -> Named Mux/18  "psi_rDot"
  GPS Vehicle State/1 -> Bus Selector/1, Map-Matching SCACS2/1(GPS Vehicle State)
  Map-Matching SCACS2/1(SCACS) -> Bus Selector1/1, Bus Selector4/1
  Bus Selector4/2 -> Named Mux/20  "<curSegProg>"
  Bus Selector4/3 -> Named Mux/21  "<e>"
  Bus Selector4/4 -> Named Mux/22  "<dPsi>"
  Bus Selector4/5 -> Named Mux/23  "<crv>"
  Bus Selector4/1 -> Named Mux/19  "<curSegType>"
  Demux/2 -> Saturation3/1  "Traction Command"
  Saturation3/1 -> Named Mux/5, Mux2/2, Mux2/1

== system DriftControllerLibrary/Driftkeeping/Enable Logic ==
  Enable Command : Inport
  Brake Pedal : Inport  Port=2
  Delay : Subsystem
  Latch1 : Subsystem  TreatAsAtomicUnit=on
  Logical Operator : Logic  Operator=OR  AllPortsSameDT=off  OutDataTypeStr=float('double')
  Logical Operator1 : Logic  AllPortsSameDT=off  OutDataTypeStr=float('double')
  Logical Operator2 : Logic  Operator=NOT  AllPortsSameDT=off  OutDataTypeStr=float('double')
  Enable : Outport
  wires:
  Latch1/1(Out1) -> Enable/1
  Enable Command/1 -> Delay/1(In), Logical Operator1/1
  Delay/1(Out) -> Logical Operator/1
  Brake Pedal/1 -> Logical Operator2/1, Logical Operator/2
  Logical Operator/1 -> Latch1/Trigger
  Logical Operator1/1 -> Latch1/1(In1)
  Logical Operator2/1 -> Logical Operator1/2

== system DriftControllerLibrary/SSC Drift Controller/Enable Logic ==
  Enable Command : Inport
  Brake Pedal : Inport  Port=2
  Delay : Subsystem
  Latch1 : Subsystem  TreatAsAtomicUnit=on
  Logical Operator : Logic  Operator=OR  AllPortsSameDT=off  OutDataTypeStr=float('double')
  Logical Operator1 : Logic  AllPortsSameDT=off  OutDataTypeStr=float('double')
  Logical Operator2 : Logic  Operator=NOT  AllPortsSameDT=off  OutDataTypeStr=float('double')
  Enable : Outport
  wires:
  Latch1/1(Out1) -> Enable/1
  Enable Command/1 -> Delay/1(In), Logical Operator1/1
  Delay/1(Out) -> Logical Operator/1
  Brake Pedal/1 -> Logical Operator2/1, Logical Operator/2
  Logical Operator/1 -> Latch1/Trigger
  Logical Operator1/1 -> Latch1/1(In1)
  Logical Operator2/1 -> Logical Operator1/2

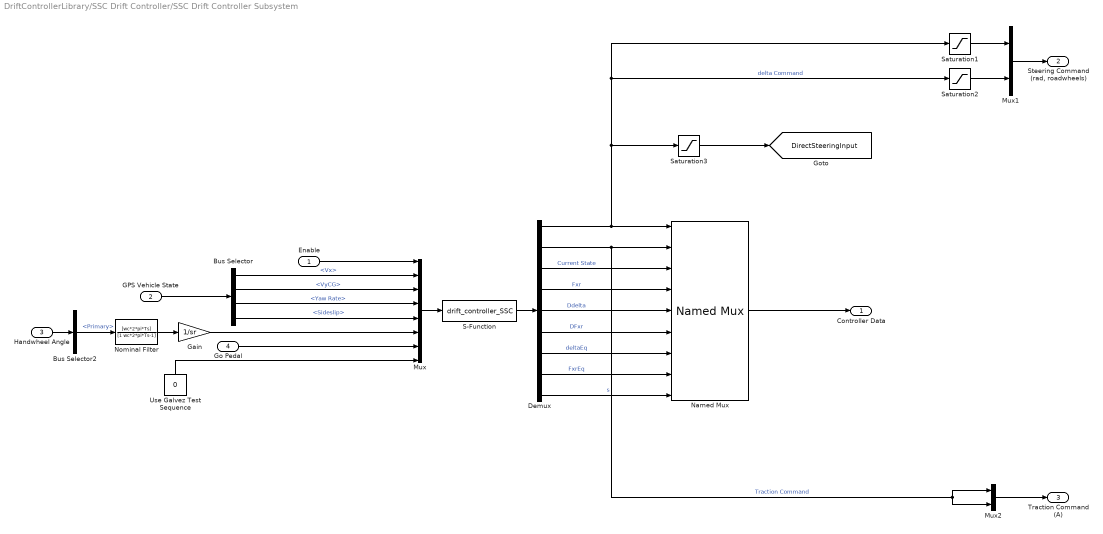
== system DriftControllerLibrary/SSC Drift Controller/SSC Drift Controller Subsystem ==
  Enable : Inport
  GPS Vehicle State : Inport  Port=2
  Handwheel Angle : Inport  Port=3
  Go Pedal : Inport  Port=4
  Bus Selector : BusSelector  OutputSignals=Vx,VyCG,Yaw Rate,Sideslip
  Bus Selector2 : BusSelector  OutputSignals=Primary
  Demux : Demux  Outputs=9
  Gain : Gain  Gain=1/sr
  Mux : Mux  Inputs=8
  Mux1 : Mux  Inputs=2
  Mux2 : Mux  Inputs=2
  Named Mux : DriftControllerLibrary/Drift Control Block/Drift Controller Subsystem/Named Mux  fname=datadescDriftControllerSSC
  Nominal Filter : DiscreteFilter  Numerator=[wc*2*pi*Ts]  Denominator=[1 wc*2*pi*Ts-1]  SampleTime=Ts
  S-Function : S-Function  FunctionName=drift_controller_SSC  Parameters=axInit,tHold,UxLimits,deltaLimits,tLimits,KUxOL,betaThreshold,rThreshold,UyEq,rEq,UxEq,deltaEq,FxrEq,mu,KUy,Kr,k11,k12,k13,k21,k22,k23,param.a, param.b, param.m, VoltsToTorque,VoltsToTorqueRegen,param.rl.r,param.drive_ratio,Ts  EnableBusSupport=off
  Saturation1 : Saturate  UpperLimit=steering_limit*pi/180  LowerLimit=-steering_limit*pi/180
  Saturation2 : Saturate  UpperLimit=steering_limit*pi/180  LowerLimit=-steering_limit*pi/180
  Saturation3 : Saturate  UpperLimit=steering_limit*pi/180  LowerLimit=-steering_limit*pi/180
  Use Galvez Test Sequence : Constant  Value=0
  Controller Data : Outport
  "Steering Command (rad, roadwheels)" : Outport  Port=2
  Traction Command (A) : Outport  Port=3
  tag scope: DirectSteeringInput=global
  wires:
  GPS Vehicle State/1 -> Bus Selector/1
  S-Function/1 -> Demux/1
  Mux/1 -> S-Function/1
  Handwheel Angle/1 -> Bus Selector2/1
  Bus Selector/1 -> Mux/2  "<Vx>"
  Enable/1 -> Mux/1
  Mux1/1 -> "Steering Command (rad, roadwheels)"/1
  Saturation1/1 -> Mux1/1
  Saturation2/1 -> Mux1/2
  Named Mux/1 -> Controller Data/1
  Bus Selector2/1 -> Nominal Filter/1  "<Primary>"
  Nominal Filter/1 -> Gain/1
  Mux2/1 -> Traction Command (A)/1
  Demux/1 -> Named Mux/1, Saturation1/1, Saturation2/1, Saturation3/1  "delta Command"
  Demux/2 -> Mux2/1, Mux2/2, Named Mux/2  "Traction Command"
  Demux/3 -> Named Mux/3  "Current State"
  Demux/4 -> Named Mux/4  "Fxr"
  Demux/5 -> Named Mux/5  "Ddelta"
  Demux/6 -> Named Mux/6  "DFxr"
  Demux/7 -> Named Mux/7  "deltaEq"
  Demux/8 -> Named Mux/8  "FxrEq"
  Demux/9 -> Named Mux/9  "s"
  Saturation3/1 -> [DirectSteeringInput]
  Bus Selector/4 -> Mux/5  "<Sideslip>"
  Gain/1 -> Mux/6
  Go Pedal/1 -> Mux/7
  Use Galvez Test Sequence/1 -> Mux/8
  Bus Selector/2 -> Mux/3  "<VyCG>"
  Bus Selector/3 -> Mux/4  "<Yaw Rate>"

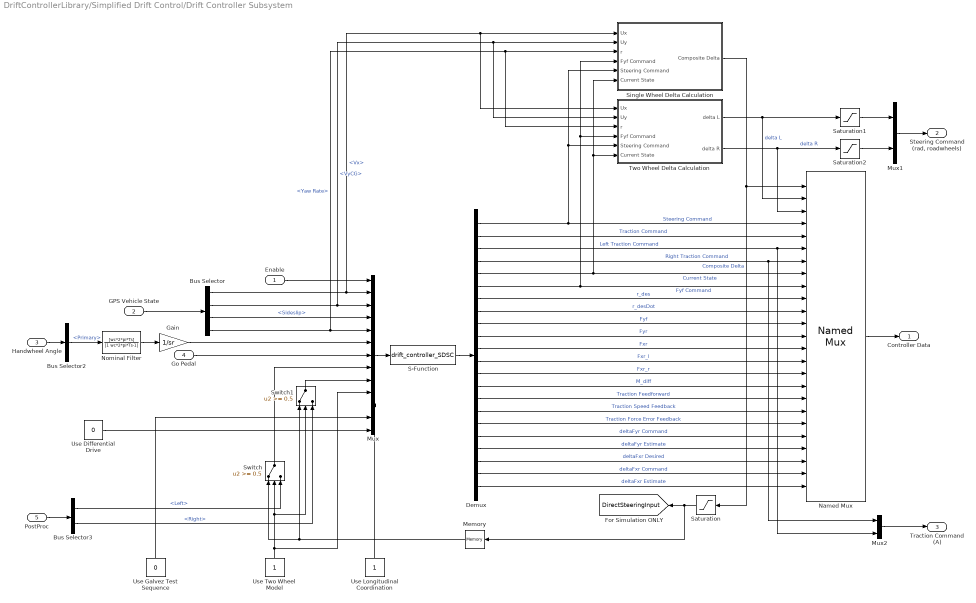
== system DriftControllerLibrary/Simplified Drift Control/Drift Controller Subsystem ==
  Enable : Inport
  GPS Vehicle State : Inport  Port=2
  Handwheel Angle : Inport  Port=3
  Go Pedal : Inport  Port=4
  PostProc : Inport  Port=5
  Bus Selector : BusSelector  OutputSignals=Vx,VyCG,Sideslip,Yaw Rate
  Bus Selector2 : BusSelector  OutputSignals=Primary
  Bus Selector3 : BusSelector  OutputSignals=Steer Angles.Left,Steer Angles.Right
  Demux : Demux  Outputs=22
  Gain : Gain  Gain=1/sr
  Memory : Memory
  Mux : Mux  Inputs=13
  Mux1 : Mux  Inputs=2
  Mux2 : Mux  Inputs=2
  Named Mux : DriftControllerLibrary/Drift Control Block/Drift Controller Subsystem/Named Mux  fname=datadescDriftControllerSDSC
  Nominal Filter : DiscreteFilter  Numerator=[wc*2*pi*Ts]  Denominator=[1 wc*2*pi*Ts-1]  SampleTime=Ts
  S-Function : S-Function  FunctionName=drift_controller_SDSC  Parameters=axInit,tHold,UxLimits,deltaLimits,tLimits,betaThreshold,rThreshold,betaDes,UxEq,FxrEq,FyfEq,FyrEq,Kbeta,Kr,KUx,KUx_Drift,VoltsToTorque,VoltsToTorqueRegen,param.drive_ratio,param.rl.r,param.m,param.Iz,param.a,param.b,param.c,param.fl.C,param.fr.C,param.rl.C,param.rr.C,mu_p_assumed,mu_s_assumed,Fyf_sat,Ts  EnableBusSupport=off
  Saturation : Saturate  UpperLimit=steering_limit*pi/180  LowerLimit=-steering_limit*pi/180
  Saturation1 : Saturate  UpperLimit=steering_limit*pi/180  LowerLimit=-steering_limit*pi/180
  Saturation2 : Saturate  UpperLimit=steering_limit*pi/180  LowerLimit=-steering_limit*pi/180
  Single Wheel Delta Calculation : Subsystem
  Switch : Switch  Threshold=0.5
  Switch1 : Switch  Threshold=0.5
  Two Wheel Delta Calculation : Subsystem
  Use Differential Drive : Constant  Value=0
  Use Galvez Test Sequence : Constant  Value=0
  Use Longitudinal Coordination : Constant
  Use Two Wheel Model : Constant
  Controller Data : Outport
  "Steering Command (rad, roadwheels)" : Outport  Port=2
  Traction Command (A) : Outport  Port=3
  tag scope: DirectSteeringInput=global
  wires:
  Mux2/1 -> Traction Command (A)/1
  Nominal Filter/1 -> Gain/1
  Bus Selector2/1 -> Nominal Filter/1  "<Primary>"
  Single Wheel Delta Calculation/1(Composite Delta) -> Saturation/1, Named Mux/1  "Composite Delta"
  Named Mux/1 -> Controller Data/1
  Two Wheel Delta Calculation/2(delta R) -> Saturation2/1, Named Mux/3  "delta R"
  Saturation2/1 -> Mux1/2
  Saturation1/1 -> Mux1/1
  Mux1/1 -> "Steering Command (rad, roadwheels)"/1
  Enable/1 -> Mux/1
  Use Galvez Test Sequence/1 -> Mux/12
  Use Longitudinal Coordination/1 -> Mux/11
  Switch1/1 -> Mux/9
  Switch/1 -> Mux/8
  Use Two Wheel Model/1 -> Switch/2, Switch1/2, Mux/10
  Bus Selector3/2 -> Switch1/3  "<Right>"
  Bus Selector3/1 -> Switch/3  "<Left>"
  Memory/1 -> Switch1/1, Switch/1
  Two Wheel Delta Calculation/1(delta L) -> Saturation1/1, Named Mux/2  "delta L"
  Saturation/1 -> Memory/1, [DirectSteeringInput]
  PostProc/1 -> Bus Selector3/1
  Bus Selector/4 -> Two Wheel Delta Calculation/3(r), Single Wheel Delta Calculation/3(r), Mux/5  "<Yaw Rate>"
  Bus Selector/3 -> Mux/4  "<Sideslip>"
  Bus Selector/2 -> Two Wheel Delta Calculation/2(Uy), Single Wheel Delta Calculation/2(Uy), Mux/3  "<VyCG>"
  Gain/1 -> Mux/6
  Go Pedal/1 -> Mux/7
  Bus Selector/1 -> Two Wheel Delta Calculation/1(Ux), Single Wheel Delta Calculation/1(Ux), Mux/2  "<Vx>"
  Handwheel Angle/1 -> Bus Selector2/1
  Mux/1 -> S-Function/1
  Use Differential Drive/1 -> Mux/13
  Demux/1 -> Single Wheel Delta Calculation/5(Steering Command), Two Wheel Delta Calculation/5(Steering Command), Named Mux/4  "Steering Command"
  Demux/2 -> Named Mux/5  "Traction Command"
  Demux/5 -> Named Mux/8, Two Wheel Delta Calculation/6(Current State), Single Wheel Delta Calculation/6(Current State)  "Current State"
  Demux/7 -> Named Mux/10  "r_des"
  Demux/6 -> Named Mux/9, Two Wheel Delta Calculation/4(Fyf Command), Single Wheel Delta Calculation/4(Fyf Command)  "Fyf Command"
  Demux/11 -> Named Mux/14  "Fxr"
  Demux/10 -> Named Mux/13  "Fyr"
  Demux/8 -> Named Mux/11  "r_desDot"
  Demux/9 -> Named Mux/12  "Fyf"
  Demux/3 -> Named Mux/6, Mux2/2  "Left Traction Command"
  Demux/4 -> Named Mux/7, Mux2/1  "Right Traction Command"
  Demux/12 -> Named Mux/15  "Fxr_l"
  Demux/13 -> Named Mux/16  "Fxr_r"
  Demux/18 -> Named Mux/21  "deltaFyr Command"
  Demux/22 -> Named Mux/25  "deltaFxr Estimate"
  Demux/21 -> Named Mux/24  "deltaFxr Command"
  Demux/20 -> Named Mux/23  "deltaFxr Desired"
  Demux/19 -> Named Mux/22  "deltaFyr Estimate"
  Demux/17 -> Named Mux/20  "Traction Force Error Feedback"
  Demux/16 -> Named Mux/19  "Traction Speed Feedback"
  Demux/15 -> Named Mux/18  "Traction Feedforward"
  Demux/14 -> Named Mux/17  "M_diff"
  S-Function/1 -> Demux/1
  GPS Vehicle State/1 -> Bus Selector/1

== system DriftControllerLibrary/Simplified Drift Control/Enable Logic ==
  Enable Command : Inport
  Brake Pedal : Inport  Port=2
  Delay : Subsystem
  Latch1 : Subsystem  TreatAsAtomicUnit=on
  Logical Operator : Logic  Operator=OR  AllPortsSameDT=off  OutDataTypeStr=float('double')
  Logical Operator1 : Logic  AllPortsSameDT=off  OutDataTypeStr=float('double')
  Logical Operator2 : Logic  Operator=NOT  AllPortsSameDT=off  OutDataTypeStr=float('double')
  Enable : Outport
  wires:
  Logical Operator2/1 -> Logical Operator1/2
  Logical Operator1/1 -> Latch1/1(In1)
  Logical Operator/1 -> Latch1/Trigger
  Brake Pedal/1 -> Logical Operator/2, Logical Operator2/1
  Delay/1(Out) -> Logical Operator/1
  Enable Command/1 -> Logical Operator1/1, Delay/1(In)
  Latch1/1(Out1) -> Enable/1

== system DriftControllerLibrary/Drift Control Block/Drift Controller Subsystem/Single Wheel Delta Calculation ==
  Ux : Inport
  Uy : Inport  Port=2
  r : Inport  Port=3
  Fyf Command : Inport  Port=4
  Steering Command : Inport  Port=5
  Current State : Inport  Port=6
  Lookup Table : Lookup  InputValues=Fyf_lookup_2W  Table=alpha_lookup  LookUpMeth=Interpolation-Use End Values
  Mux1 : Mux  Inputs=3
  "Slip Angle " : Fcn  Expr=atan2(u[2] + param.a*u[3], u[1])*(u[1] >= 0.5)
  Sum : Sum  Inputs=+-|
  Switch : Switch  Threshold=4.5
  Composite Delta : Outport
  wires:
  Switch/1 -> Composite Delta/1
  r/1 -> Mux1/3
  Uy/1 -> Mux1/2
  Ux/1 -> Mux1/1
  Fyf Command/1 -> Lookup Table/1
  Current State/1 -> Switch/2
  Steering Command/1 -> Switch/3
  Sum/1 -> Switch/1
  "Slip Angle "/1 -> Sum/1
  Lookup Table/1 -> Sum/2
  Mux1/1 -> "Slip Angle "/1

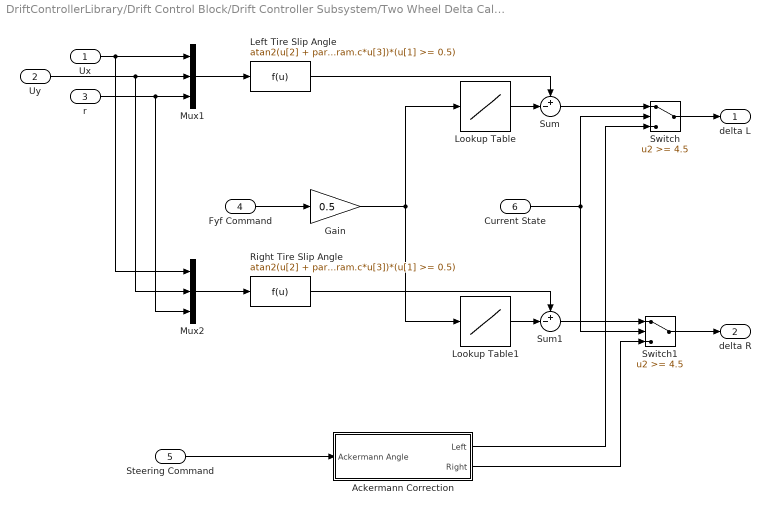
== system DriftControllerLibrary/Drift Control Block/Drift Controller Subsystem/Two Wheel Delta Calculation ==
  Ux : Inport
  Uy : Inport  Port=2
  r : Inport  Port=3
  Fyf Command : Inport  Port=4
  Steering Command : Inport  Port=5
  Current State : Inport  Port=6
  Ackermann Correction : Subsystem
  Gain : Gain  Gain=0.5
  Left Tire Slip Angle : Fcn  Expr=atan2(u[2] + param.a*u[3], u[1]-param.c*u[3])*(u[1] >= 0.5)
  Lookup Table : Lookup  InputValues=Fyf_lookup_4W  Table=alpha_lookup  LookUpMeth=Interpolation-Use End Values
  Lookup Table1 : Lookup  InputValues=Fyf_lookup_4W  Table=alpha_lookup  LookUpMeth=Interpolation-Use End Values
  Mux1 : Mux  Inputs=3
  Mux2 : Mux  Inputs=3
  Right Tire Slip Angle : Fcn  Expr=atan2(u[2] + param.a*u[3], u[1]+param.c*u[3])*(u[1] >= 0.5)
  Sum : Sum  Inputs=+-|
  Sum1 : Sum  Inputs=+-|
  Switch : Switch  Threshold=4.5
  Switch1 : Switch  Threshold=4.5
  delta L : Outport
  delta R : Outport  Port=2
  wires:
  Ackermann Correction/2(Right) -> Switch1/3
  Ackermann Correction/1(Left) -> Switch/3
  Steering Command/1 -> Ackermann Correction/1(Ackermann Angle)
  Current State/1 -> Switch1/2, Switch/2
  Sum1/1 -> Switch1/1
  Switch1/1 -> delta R/1
  Right Tire Slip Angle/1 -> Sum1/1
  Lookup Table1/1 -> Sum1/2
  Gain/1 -> Lookup Table1/1, Lookup Table/1
  Fyf Command/1 -> Gain/1
  Mux2/1 -> Right Tire Slip Angle/1
  Switch/1 -> delta L/1
  r/1 -> Mux2/3, Mux1/3
  Uy/1 -> Mux2/2, Mux1/2
  Ux/1 -> Mux2/1, Mux1/1
  Sum/1 -> Switch/1
  Left Tire Slip Angle/1 -> Sum/1
  Lookup Table/1 -> Sum/2
  Mux1/1 -> Left Tire Slip Angle/1

== system DriftControllerLibrary/Drift Control Block/Enable Logic/Delay ==
  In : Inport
  Unit Delay{,1..4} (5 alike) : UnitDelay  SampleTime=Ts
  Out : Outport
  wires:
  Unit Delay4/1 -> Out/1
  Unit Delay3/1 -> Unit Delay4/1
  Unit Delay2/1 -> Unit Delay3/1
  Unit Delay1/1 -> Unit Delay2/1
  Unit Delay/1 -> Unit Delay1/1
  In/1 -> Unit Delay/1

== system DriftControllerLibrary/Drift Control Block/Enable Logic/Latch1 ==
  In1 : Inport
  Trigger : TriggerPort
  Out1 : Outport  InitialOutput=0
  wires:
  In1/1 -> Out1/1
